simulink model "PLANT_MODEL"  (R2021b)
settings: Solver=FixedStepAuto  StartTime=0.0  StopTime=20.0  FixedStep=0.01  RelTol=1e-3
PreLoadFcn:
  | run('MAIN.m');
values from neighbouring files (symbols this model uses):
  uFB0 = [delta_r; lambdas0_w]    [MAIN.m]
  x0 = 0    [ESP_main.m]    (also in EigenValuesLocus.m = [v0; 0; 0]; MAIN.m = [0; 0; v0; 0; 0; 0])
settings Model: Creator=atavo  LastModifiedBy=atavo

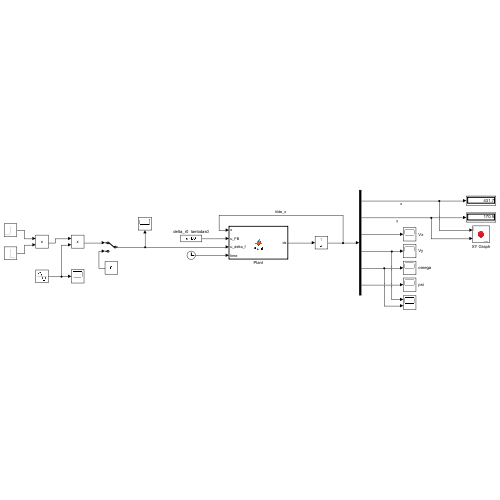
[thumbnail: Simulink's stored preview of the top-level diagram]
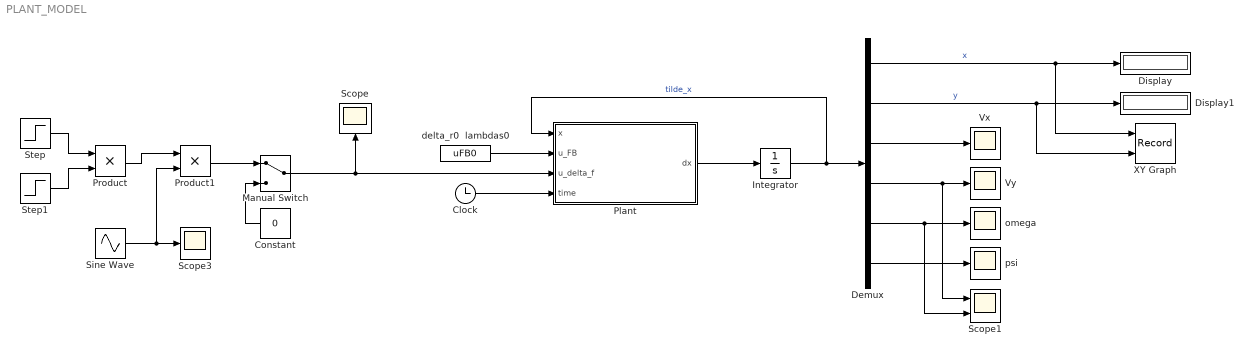
== system PLANT_MODEL ==
  Clock : Clock
      settings: Decimation=1000
  Constant : Constant  Value=0
  Demux : Demux  Outputs=6
  Display : Display
  Display1 : Display
  Integrator : Integrator  InitialCondition=x0
  Manual Switch : ManualSwitch
  Plant : MATLAB Function  TreatAsAtomicUnit=on
  Product : Product
  Product1 : Product
  Scope : Scope
  Scope1 : Scope  NumInputPorts=2
  Scope3 : Scope
  Sine Wave : Sin  Amplitude=5*(pi/180)  Frequency=pi  Phase=-3*pi  SampleTime=0
  Step : Step  Time=3  SampleTime=0
  Step1 : Step  Time=5  Before=1  After=0  SampleTime=0
  Vx : Scope
  Vy : Scope
  XY Graph : Record  FileSettingsInternal="{\"entries\":[{\"content\":{\"excelSettings\":{\"content\":{},\"type\":\"Streamout.ExcelSettings\"}},\"type\":\"Streamout.FileSettingStorage\",\"uuid\":\"16877428-a5cd-4751-a5d1-7bad0c5bb4b0\"}],\"packageUris\":[\"http://schema.mathworks.com/mf0/streamout_blocks/R2020a\"],\"version\":\"1.0\"}"  Layout=[1 1]  SignalsInternal="{\"entries\":[{\"content\":{\"signals\":[{\"content\":{\"blockPath\":[\"PLANT_MODEL/XY Graph\"],\"channel\":[],\"dimensions\":[1],\"domain\":\"PLANT_MODEL/XY Graph\",\"lineColor\":\"#a2142f\",\"plots\":[1],\"port\":1,\"sid\":[\"\"],\"signalID\":1211,\"signalName\":\"x\"},\"type\":\"RecordBlkView.Signal\",\"uuid\":\"a5f8ff9e-ce7b-42f5-83f4-a8a19ac39355\"},{\"content\":{\"blockPath\":[\"PLANT_MODEL/XY Graph\"],\"channel\":[],\"dimensions\":[1],\"domain\":\"PLANT_MODEL/XY Graph\",\"lineColor\":\"#139fff\",\"plots\":[1],\"port\":2,\"sid\":[\"\"],\"signalID\":1215,\"signalName\":\"y\"},\"type\":\"RecordBlkView.Signal\",\"uuid\":\"423f0ca2-8831-441e-98a3-233246c0cf8a\"}]},\"type\":\"RecordBlkView.InputSignals\",\"uuid\":\"1a689944-4edf-4764-9c9f-996dbe819701\"}],\"packageUris\":[\"http://schema.mathworks.com/mf0/streamout_blocks/R2020a\"],\"version\":\"1.0\"}"  VisualizationBindings="{\"xyplotplugin\":{\"info\":[{\"series\":[{\"bindingParametersList\":[{\"parameter\":\"X-Axis\",\"signalID\":1211,\"signalName\":\"x\"},{\"parameter\":\"Y-Axis\",\"signalID\":1215,\"signalName\":\"y\"}],\"seriesID\":39792}],\"subplotID\":1}]}}"  CompatibilityTag=XY  st=-1
  delta_r0  lambdas0 : Constant  Value=uFB0
  omega : Scope
  psi : Scope
  wires:
  Plant/1(dx) -> Integrator/1
  delta_r0  lambdas0/1 -> Plant/2(u_FB)
  Integrator/1 -> Plant/1(x), Demux/1  "tilde_x"
  Step/1 -> Product/1
  Demux/1 -> XY Graph/1, Display/1  "x"
  Demux/2 -> XY Graph/2, Display1/1  "y"
  Demux/3 -> Vx/1
  Demux/4 -> Scope1/1, Vy/1
  Demux/5 -> Scope1/2, omega/1
  Demux/6 -> psi/1
  Clock/1 -> Plant/4(time)
  Step1/1 -> Product/2
  Manual Switch/1 -> Plant/3(u_delta_f), Scope/1
  Sine Wave/1 -> Scope3/1, Product1/2
  Product/1 -> Product1/1
  Product1/1 -> Manual Switch/1
  Constant/1 -> Manual Switch/2

== matlab function PLANT_MODEL/Plant ==
  data: x input; dx output; u_FB input; u_delta_f input; time input
function dx = Plant(x,u_FB,u_delta_f, time)
    % ridefinisco dentro il plant tutte le costanti che mi servono
    %global rho S v0 Cx N_wheels CR
    %global g Cy rk r_x r_y r_z m J
    
    g   = 9.81;                         % [m/s^2] gravity acceleration
    rho = 1.225;                        % [kg/m^3] air density
    Cx  = 0.3;                          % drag coefficient 
    Cy  = 0.3;                          % drag coefficient
    rk  = 1;                            % dry asphalt
    
    r_x = [1.6 1.6 -1.4 -1.4];
    r_y = [0.9 -0.9 0.9 -0.9];
    r_z = 0.70;
    S   = 2.4;                          % [m^2] cross surface
    m   = 1200;                         % [kg] vehicle mass
    J   = m*(r_x(4)^2+r_y(1)^2)^2;      % Vehicle inertia
    
    CR = 0.05;                          % coefficiente attrito resistenza delle ruote
    
   
    if(time>5)
        disp(time);
    end
    % le condizioni iniziali le metto dentro l'integratore, il plant è non
    % lineare quindi non devo sommare x0 perchè non ho realizzato un
    % quanlche controllo su di lui
    posin_x     = x(1);
    posin_y     = x(2);
    v_x_body    = x(3); 
    v_y_body    = x(4);
    omega       = x(5); % yaw angular speed
    psi         = x(6); % yaw angle
    
    %NL plant vuole 4 lambda, la soluzione del problema di controllo
    %ottimale nel MAIN è fatta con u_eq, ricostruiamo poi 1 4 u_lambda
    u_delta_r = u_FB(1);
    lambdas = zeros(1,4);
    lambdas(1) = u_FB(2);
    lambdas(2) = u_FB(3);
    lambdas(3) = u_FB(4);
    lambdas(4) = u_FB(5);
    
    delta_w = zeros(1,4);
    delta_w(1) = u_delta_f;
    delta_w(2) = u_delta_f;
    delta_w(3) = u_delta_r;
    delta_w(4) = u_delta_r;
    
    
    
    AeroForce   = 0.5*rho*S *[(v_x_body^2)*Cx
                              (v_y_body^2)*Cy];

    mu_body     = zeros(2,4);
    f_x_wheels  = zeros(1,4);
    f_y_wheels  = zeros(1,4);

for i = 1:4

    Rot_btowi        = [cos(delta_w(i)) sin(delta_w(i));
                       -sin(delta_w(i)) cos(delta_w(i))];
    
    v_wheeli        = Rot_btowi*([-omega*r_y(i) ; omega*r_x(i)] + [v_x_body ; v_y_body]);
    
    beta_wheeli      = atan(v_wheeli(2)/v_wheeli(1));
   
    mu_lambdai       = mu_long(rk, lambdas(i));                                 % Dry asphalt
    mu_betai         = mu_long(rk, beta_wheeli);                                 % Dry asphalt
    
    mu_body(1,i)    = mu_lambdai;
    mu_body(2,i)    = mu_betai;
    
end
    
    N               = m*g;
    
    H               = [ones(1,4)
                        -r_x
                         r_y   ];

    N_wheels        = [3320.6;3320.6;2364.8;2364.8];
    
%     N_wheels        = pinv(H) * [         N
%                                   0.5*rho*(v_x_body^2)*S*Cx*r_z
%                                           0                ];
f_x = 0;
f_y = 0;
tau = 0;
for i = 1:4
    f_x_wheels(i) = + N_wheels(i)*mu_body(1,i);
    f_y_wheels(i) = - N_wheels(i)*mu_body(2,i);

    f_x     = f_x + (cos(delta_w(i))*f_x_wheels(i) -sin(delta_w(i))*f_y_wheels(i));
    f_y     = f_y + (sin(delta_w(i))*f_x_wheels(i) +cos(delta_w(i))*f_y_wheels(i));
    tau     = tau + (sin(delta_w(i))*f_y_wheels(i) -cos(delta_w(i))*f_x_wheels(i))*r_y(i) + (sin(delta_w(i))*f_x_wheels(i) +cos(delta_w(i))*f_y_wheels(i))*r_x(i);
end 


dv_x_body        = (f_x + (m*omega*v_y_body) - (0.5*rho*S*(v_x_body^2)*Cx))/m;
dv_y_body        = (f_y - (m*omega*v_x_body))/m;
domega           = tau/J;
dpsi             = omega;

[beta,v] = cart2pol(v_x_body,v_y_body);

dx          = [v*cos(psi+beta);
               v*sin(psi+beta);
               dv_x_body*0; % ricordare che imponiamo la v_x costante, ha senso mettere quindi questo a zero così?
               dv_y_body;
               domega;
               dpsi];                                                     

           

end

function mu = mu_long(i,lambda) %12.1d

% 1) Dry asphalt
% 2) wet asphalt
% 3) Snow
% 4) Ice
% 5) Dry Cobblestone
% 6) wet cobblestone
theta1 = [1.28 0.86 0.19 0.05 1.37 0.4];
theta2 = [23.99 33.82 94.13 306.39 6.46 33.71];
theta3 = [0.52 0.35 0.05 0 0.67 0.12];

mu = sign(lambda).*theta1(i).*(1-exp(-abs(lambda)*theta2(i)))-theta3(i)*lambda;
end
